simulink model "signal_tranmission"  (R2024b)
settings: Solver=ode45  StartTime=0.0  StopTime=10  FixedStep=0.000125  RelTol=1e-3
libraries: dspfdesign x500, commchan3 x1
(part 6 of 7)

== system signal_tranmission/SSB Modulator21/Balanced Modulator ==
  note: -S2(t)
  note: S1(t)
  note: -m(t)
  note: m(t)
  note: S2(t)
  note: S1(t)
  Input Signal : Inport
  Carrier Signal : Inport  Port=2
  -S2(t) : Product
  Add : Sum
  Add1 : Sum
  Add2 : Sum
  Constant : Constant
  Constant1 : Constant  Value=-1
  Constant2 : Constant
  Constant3 : Constant  Value=-1
  Product1 : Product
  S1(t) : Product
  S2(t) : Product
  DSBSC : Outport
  wires:
  Product1/1 -> Add1/1
  Add/1 -> S1(t)/1
  Constant3/1 -> -S2(t)/2
  Constant2/1 -> Add1/2
  S2(t)/1 -> -S2(t)/1
  Carrier Signal/1 -> S1(t)/2, S2(t)/1
  Constant/1 -> Add/2
  Add1/1 -> S2(t)/2
  Constant1/1 -> Product1/2
  -S2(t)/1 -> Add2/2
  S1(t)/1 -> Add2/1
  Input Signal/1 -> Product1/1, Add/1
  Add2/1 -> DSBSC/1

== system signal_tranmission/SSB Modulator22/Balanced Modulator ==
  note: -S2(t)
  note: S1(t)
  note: -m(t)
  note: m(t)
  note: S2(t)
  note: S1(t)
  Input Signal : Inport
  Carrier Signal : Inport  Port=2
  -S2(t) : Product
  Add : Sum
  Add1 : Sum
  Add2 : Sum
  Constant : Constant
  Constant1 : Constant  Value=-1
  Constant2 : Constant
  Constant3 : Constant  Value=-1
  Product1 : Product
  S1(t) : Product
  S2(t) : Product
  DSBSC : Outport
  wires:
  Product1/1 -> Add1/1
  Add/1 -> S1(t)/1
  Constant3/1 -> -S2(t)/2
  Constant2/1 -> Add1/2
  S2(t)/1 -> -S2(t)/1
  Carrier Signal/1 -> S1(t)/2, S2(t)/1
  Constant/1 -> Add/2
  Add1/1 -> S2(t)/2
  Constant1/1 -> Product1/2
  -S2(t)/1 -> Add2/2
  S1(t)/1 -> Add2/1
  Input Signal/1 -> Product1/1, Add/1
  Add2/1 -> DSBSC/1

== system signal_tranmission/SSB Modulator23/Balanced Modulator ==
  note: -S2(t)
  note: S1(t)
  note: -m(t)
  note: m(t)
  note: S2(t)
  note: S1(t)
  Input Signal : Inport
  Carrier Signal : Inport  Port=2
  -S2(t) : Product
  Add : Sum
  Add1 : Sum
  Add2 : Sum
  Constant : Constant
  Constant1 : Constant  Value=-1
  Constant2 : Constant
  Constant3 : Constant  Value=-1
  Product1 : Product
  S1(t) : Product
  S2(t) : Product
  DSBSC : Outport
  wires:
  Product1/1 -> Add1/1
  Add/1 -> S1(t)/1
  Constant3/1 -> -S2(t)/2
  Constant2/1 -> Add1/2
  S2(t)/1 -> -S2(t)/1
  Carrier Signal/1 -> S1(t)/2, S2(t)/1
  Constant/1 -> Add/2
  Add1/1 -> S2(t)/2
  Constant1/1 -> Product1/2
  -S2(t)/1 -> Add2/2
  S1(t)/1 -> Add2/1
  Input Signal/1 -> Product1/1, Add/1
  Add2/1 -> DSBSC/1

== system signal_tranmission/SSB Modulator24/Balanced Modulator ==
  note: -S2(t)
  note: S1(t)
  note: -m(t)
  note: m(t)
  note: S2(t)
  note: S1(t)
  Input Signal : Inport
  Carrier Signal : Inport  Port=2
  -S2(t) : Product
  Add : Sum
  Add1 : Sum
  Add2 : Sum
  Constant : Constant
  Constant1 : Constant  Value=-1
  Constant2 : Constant
  Constant3 : Constant  Value=-1
  Product1 : Product
  S1(t) : Product
  S2(t) : Product
  DSBSC : Outport
  wires:
  Product1/1 -> Add1/1
  Add/1 -> S1(t)/1
  Constant3/1 -> -S2(t)/2
  Constant2/1 -> Add1/2
  S2(t)/1 -> -S2(t)/1
  Carrier Signal/1 -> S1(t)/2, S2(t)/1
  Constant/1 -> Add/2
  Add1/1 -> S2(t)/2
  Constant1/1 -> Product1/2
  -S2(t)/1 -> Add2/2
  S1(t)/1 -> Add2/1
  Input Signal/1 -> Product1/1, Add/1
  Add2/1 -> DSBSC/1

== system signal_tranmission/SSB Modulator25/Balanced Modulator ==
  note: -S2(t)
  note: S1(t)
  note: -m(t)
  note: m(t)
  note: S2(t)
  note: S1(t)
  Input Signal : Inport
  Carrier Signal : Inport  Port=2
  -S2(t) : Product
  Add : Sum
  Add1 : Sum
  Add2 : Sum
  Constant : Constant
  Constant1 : Constant  Value=-1
  Constant2 : Constant
  Constant3 : Constant  Value=-1
  Product1 : Product
  S1(t) : Product
  S2(t) : Product
  DSBSC : Outport
  wires:
  Product1/1 -> Add1/1
  Add/1 -> S1(t)/1
  Constant3/1 -> -S2(t)/2
  Constant2/1 -> Add1/2
  S2(t)/1 -> -S2(t)/1
  Carrier Signal/1 -> S1(t)/2, S2(t)/1
  Constant/1 -> Add/2
  Add1/1 -> S2(t)/2
  Constant1/1 -> Product1/2
  -S2(t)/1 -> Add2/2
  S1(t)/1 -> Add2/1
  Input Signal/1 -> Product1/1, Add/1
  Add2/1 -> DSBSC/1

== system signal_tranmission/SSB Modulator26/Balanced Modulator ==
  note: -S2(t)
  note: S1(t)
  note: -m(t)
  note: m(t)
  note: S2(t)
  note: S1(t)
  Input Signal : Inport
  Carrier Signal : Inport  Port=2
  -S2(t) : Product
  Add : Sum
  Add1 : Sum
  Add2 : Sum
  Constant : Constant
  Constant1 : Constant  Value=-1
  Constant2 : Constant
  Constant3 : Constant  Value=-1
  Product1 : Product
  S1(t) : Product
  S2(t) : Product
  DSBSC : Outport
  wires:
  Product1/1 -> Add1/1
  Add/1 -> S1(t)/1
  Constant3/1 -> -S2(t)/2
  Constant2/1 -> Add1/2
  S2(t)/1 -> -S2(t)/1
  Carrier Signal/1 -> S1(t)/2, S2(t)/1
  Constant/1 -> Add/2
  Add1/1 -> S2(t)/2
  Constant1/1 -> Product1/2
  -S2(t)/1 -> Add2/2
  S1(t)/1 -> Add2/1
  Input Signal/1 -> Product1/1, Add/1
  Add2/1 -> DSBSC/1

== system signal_tranmission/SSB Modulator27/Balanced Modulator ==
  note: -S2(t)
  note: S1(t)
  note: -m(t)
  note: m(t)
  note: S2(t)
  note: S1(t)
  Input Signal : Inport
  Carrier Signal : Inport  Port=2
  -S2(t) : Product
  Add : Sum
  Add1 : Sum
  Add2 : Sum
  Constant : Constant
  Constant1 : Constant  Value=-1
  Constant2 : Constant
  Constant3 : Constant  Value=-1
  Product1 : Product
  S1(t) : Product
  S2(t) : Product
  DSBSC : Outport
  wires:
  Product1/1 -> Add1/1
  Add/1 -> S1(t)/1
  Constant3/1 -> -S2(t)/2
  Constant2/1 -> Add1/2
  S2(t)/1 -> -S2(t)/1
  Carrier Signal/1 -> S1(t)/2, S2(t)/1
  Constant/1 -> Add/2
  Add1/1 -> S2(t)/2
  Constant1/1 -> Product1/2
  -S2(t)/1 -> Add2/2
  S1(t)/1 -> Add2/1
  Input Signal/1 -> Product1/1, Add/1
  Add2/1 -> DSBSC/1

== system signal_tranmission/SSB Modulator28/Balanced Modulator ==
  note: -S2(t)
  note: S1(t)
  note: -m(t)
  note: m(t)
  note: S2(t)
  note: S1(t)
  Input Signal : Inport
  Carrier Signal : Inport  Port=2
  -S2(t) : Product
  Add : Sum
  Add1 : Sum
  Add2 : Sum
  Constant : Constant
  Constant1 : Constant  Value=-1
  Constant2 : Constant
  Constant3 : Constant  Value=-1
  Product1 : Product
  S1(t) : Product
  S2(t) : Product
  DSBSC : Outport
  wires:
  Product1/1 -> Add1/1
  Add/1 -> S1(t)/1
  Constant3/1 -> -S2(t)/2
  Constant2/1 -> Add1/2
  S2(t)/1 -> -S2(t)/1
  Carrier Signal/1 -> S1(t)/2, S2(t)/1
  Constant/1 -> Add/2
  Add1/1 -> S2(t)/2
  Constant1/1 -> Product1/2
  -S2(t)/1 -> Add2/2
  S1(t)/1 -> Add2/1
  Input Signal/1 -> Product1/1, Add/1
  Add2/1 -> DSBSC/1

== system signal_tranmission/SSB Modulator29/Balanced Modulator ==
  note: -S2(t)
  note: S1(t)
  note: -m(t)
  note: m(t)
  note: S2(t)
  note: S1(t)
  Input Signal : Inport
  Carrier Signal : Inport  Port=2
  -S2(t) : Product
  Add : Sum
  Add1 : Sum
  Add2 : Sum
  Constant : Constant
  Constant1 : Constant  Value=-1
  Constant2 : Constant
  Constant3 : Constant  Value=-1
  Product1 : Product
  S1(t) : Product
  S2(t) : Product
  DSBSC : Outport
  wires:
  Product1/1 -> Add1/1
  Add/1 -> S1(t)/1
  Constant3/1 -> -S2(t)/2
  Constant2/1 -> Add1/2
  S2(t)/1 -> -S2(t)/1
  Carrier Signal/1 -> S1(t)/2, S2(t)/1
  Constant/1 -> Add/2
  Add1/1 -> S2(t)/2
  Constant1/1 -> Product1/2
  -S2(t)/1 -> Add2/2
  S1(t)/1 -> Add2/1
  Input Signal/1 -> Product1/1, Add/1
  Add2/1 -> DSBSC/1

== system signal_tranmission/SSB Modulator3/Balanced Modulator ==
  note: -S2(t)
  note: S1(t)
  note: -m(t)
  note: m(t)
  note: S2(t)
  note: S1(t)
  Input Signal : Inport
  Carrier Signal : Inport  Port=2
  -S2(t) : Product
  Add : Sum
  Add1 : Sum
  Add2 : Sum
  Constant : Constant
  Constant1 : Constant  Value=-1
  Constant2 : Constant
  Constant3 : Constant  Value=-1
  Product1 : Product
  S1(t) : Product
  S2(t) : Product
  DSBSC : Outport
  wires:
  Product1/1 -> Add1/1
  Add/1 -> S1(t)/1
  Constant3/1 -> -S2(t)/2
  Constant2/1 -> Add1/2
  S2(t)/1 -> -S2(t)/1
  Carrier Signal/1 -> S1(t)/2, S2(t)/1
  Constant/1 -> Add/2
  Add1/1 -> S2(t)/2
  Constant1/1 -> Product1/2
  -S2(t)/1 -> Add2/2
  S1(t)/1 -> Add2/1
  Input Signal/1 -> Product1/1, Add/1
  Add2/1 -> DSBSC/1

== system signal_tranmission/SSB Modulator30/Balanced Modulator ==
  note: -S2(t)
  note: S1(t)
  note: -m(t)
  note: m(t)
  note: S2(t)
  note: S1(t)
  Input Signal : Inport
  Carrier Signal : Inport  Port=2
  -S2(t) : Product
  Add : Sum
  Add1 : Sum
  Add2 : Sum
  Constant : Constant
  Constant1 : Constant  Value=-1
  Constant2 : Constant
  Constant3 : Constant  Value=-1
  Product1 : Product
  S1(t) : Product
  S2(t) : Product
  DSBSC : Outport
  wires:
  Product1/1 -> Add1/1
  Add/1 -> S1(t)/1
  Constant3/1 -> -S2(t)/2
  Constant2/1 -> Add1/2
  S2(t)/1 -> -S2(t)/1
  Carrier Signal/1 -> S1(t)/2, S2(t)/1
  Constant/1 -> Add/2
  Add1/1 -> S2(t)/2
  Constant1/1 -> Product1/2
  -S2(t)/1 -> Add2/2
  S1(t)/1 -> Add2/1
  Input Signal/1 -> Product1/1, Add/1
  Add2/1 -> DSBSC/1

== system signal_tranmission/SSB Modulator31/Balanced Modulator ==
  note: -S2(t)
  note: S1(t)
  note: -m(t)
  note: m(t)
  note: S2(t)
  note: S1(t)
  Input Signal : Inport
  Carrier Signal : Inport  Port=2
  -S2(t) : Product
  Add : Sum
  Add1 : Sum
  Add2 : Sum
  Constant : Constant
  Constant1 : Constant  Value=-1
  Constant2 : Constant
  Constant3 : Constant  Value=-1
  Product1 : Product
  S1(t) : Product
  S2(t) : Product
  DSBSC : Outport
  wires:
  Product1/1 -> Add1/1
  Add/1 -> S1(t)/1
  Constant3/1 -> -S2(t)/2
  Constant2/1 -> Add1/2
  S2(t)/1 -> -S2(t)/1
  Carrier Signal/1 -> S1(t)/2, S2(t)/1
  Constant/1 -> Add/2
  Add1/1 -> S2(t)/2
  Constant1/1 -> Product1/2
  -S2(t)/1 -> Add2/2
  S1(t)/1 -> Add2/1
  Input Signal/1 -> Product1/1, Add/1
  Add2/1 -> DSBSC/1

== system signal_tranmission/SSB Modulator32/Balanced Modulator ==
  note: -S2(t)
  note: S1(t)
  note: -m(t)
  note: m(t)
  note: S2(t)
  note: S1(t)
  Input Signal : Inport
  Carrier Signal : Inport  Port=2
  -S2(t) : Product
  Add : Sum
  Add1 : Sum
  Add2 : Sum
  Constant : Constant
  Constant1 : Constant  Value=-1
  Constant2 : Constant
  Constant3 : Constant  Value=-1
  Product1 : Product
  S1(t) : Product
  S2(t) : Product
  DSBSC : Outport
  wires:
  Product1/1 -> Add1/1
  Add/1 -> S1(t)/1
  Constant3/1 -> -S2(t)/2
  Constant2/1 -> Add1/2
  S2(t)/1 -> -S2(t)/1
  Carrier Signal/1 -> S1(t)/2, S2(t)/1
  Constant/1 -> Add/2
  Add1/1 -> S2(t)/2
  Constant1/1 -> Product1/2
  -S2(t)/1 -> Add2/2
  S1(t)/1 -> Add2/1
  Input Signal/1 -> Product1/1, Add/1
  Add2/1 -> DSBSC/1

== system signal_tranmission/SSB Modulator33/Balanced Modulator ==
  note: -S2(t)
  note: S1(t)
  note: -m(t)
  note: m(t)
  note: S2(t)
  note: S1(t)
  Input Signal : Inport
  Carrier Signal : Inport  Port=2
  -S2(t) : Product
  Add : Sum
  Add1 : Sum
  Add2 : Sum
  Constant : Constant
  Constant1 : Constant  Value=-1
  Constant2 : Constant
  Constant3 : Constant  Value=-1
  Product1 : Product
  S1(t) : Product
  S2(t) : Product
  DSBSC : Outport
  wires:
  Product1/1 -> Add1/1
  Add/1 -> S1(t)/1
  Constant3/1 -> -S2(t)/2
  Constant2/1 -> Add1/2
  S2(t)/1 -> -S2(t)/1
  Carrier Signal/1 -> S1(t)/2, S2(t)/1
  Constant/1 -> Add/2
  Add1/1 -> S2(t)/2
  Constant1/1 -> Product1/2
  -S2(t)/1 -> Add2/2
  S1(t)/1 -> Add2/1
  Input Signal/1 -> Product1/1, Add/1
  Add2/1 -> DSBSC/1

== system signal_tranmission/SSB Modulator34/Balanced Modulator ==
  note: -S2(t)
  note: S1(t)
  note: -m(t)
  note: m(t)
  note: S2(t)
  note: S1(t)
  Input Signal : Inport
  Carrier Signal : Inport  Port=2
  -S2(t) : Product
  Add : Sum
  Add1 : Sum
  Add2 : Sum
  Constant : Constant
  Constant1 : Constant  Value=-1
  Constant2 : Constant
  Constant3 : Constant  Value=-1
  Product1 : Product
  S1(t) : Product
  S2(t) : Product
  DSBSC : Outport
  wires:
  Product1/1 -> Add1/1
  Add/1 -> S1(t)/1
  Constant3/1 -> -S2(t)/2
  Constant2/1 -> Add1/2
  S2(t)/1 -> -S2(t)/1
  Carrier Signal/1 -> S1(t)/2, S2(t)/1
  Constant/1 -> Add/2
  Add1/1 -> S2(t)/2
  Constant1/1 -> Product1/2
  -S2(t)/1 -> Add2/2
  S1(t)/1 -> Add2/1
  Input Signal/1 -> Product1/1, Add/1
  Add2/1 -> DSBSC/1

== system signal_tranmission/SSB Modulator35/Balanced Modulator ==
  note: -S2(t)
  note: S1(t)
  note: -m(t)
  note: m(t)
  note: S2(t)
  note: S1(t)
  Input Signal : Inport
  Carrier Signal : Inport  Port=2
  -S2(t) : Product
  Add : Sum
  Add1 : Sum
  Add2 : Sum
  Constant : Constant
  Constant1 : Constant  Value=-1
  Constant2 : Constant
  Constant3 : Constant  Value=-1
  Product1 : Product
  S1(t) : Product
  S2(t) : Product
  DSBSC : Outport
  wires:
  Product1/1 -> Add1/1
  Add/1 -> S1(t)/1
  Constant3/1 -> -S2(t)/2
  Constant2/1 -> Add1/2
  S2(t)/1 -> -S2(t)/1
  Carrier Signal/1 -> S1(t)/2, S2(t)/1
  Constant/1 -> Add/2
  Add1/1 -> S2(t)/2
  Constant1/1 -> Product1/2
  -S2(t)/1 -> Add2/2
  S1(t)/1 -> Add2/1
  Input Signal/1 -> Product1/1, Add/1
  Add2/1 -> DSBSC/1

== system signal_tranmission/SSB Modulator36/Balanced Modulator ==
  note: -S2(t)
  note: S1(t)
  note: -m(t)
  note: m(t)
  note: S2(t)
  note: S1(t)
  Input Signal : Inport
  Carrier Signal : Inport  Port=2
  -S2(t) : Product
  Add : Sum
  Add1 : Sum
  Add2 : Sum
  Constant : Constant
  Constant1 : Constant  Value=-1
  Constant2 : Constant
  Constant3 : Constant  Value=-1
  Product1 : Product
  S1(t) : Product
  S2(t) : Product
  DSBSC : Outport
  wires:
  Product1/1 -> Add1/1
  Add/1 -> S1(t)/1
  Constant3/1 -> -S2(t)/2
  Constant2/1 -> Add1/2
  S2(t)/1 -> -S2(t)/1
  Carrier Signal/1 -> S1(t)/2, S2(t)/1
  Constant/1 -> Add/2
  Add1/1 -> S2(t)/2
  Constant1/1 -> Product1/2
  -S2(t)/1 -> Add2/2
  S1(t)/1 -> Add2/1
  Input Signal/1 -> Product1/1, Add/1
  Add2/1 -> DSBSC/1

== system signal_tranmission/SSB Modulator37/Balanced Modulator ==
  note: -S2(t)
  note: S1(t)
  note: -m(t)
  note: m(t)
  note: S2(t)
  note: S1(t)
  Input Signal : Inport
  Carrier Signal : Inport  Port=2
  -S2(t) : Product
  Add : Sum
  Add1 : Sum
  Add2 : Sum
  Constant : Constant
  Constant1 : Constant  Value=-1
  Constant2 : Constant
  Constant3 : Constant  Value=-1
  Product1 : Product
  S1(t) : Product
  S2(t) : Product
  DSBSC : Outport
  wires:
  Product1/1 -> Add1/1
  Add/1 -> S1(t)/1
  Constant3/1 -> -S2(t)/2
  Constant2/1 -> Add1/2
  S2(t)/1 -> -S2(t)/1
  Carrier Signal/1 -> S1(t)/2, S2(t)/1
  Constant/1 -> Add/2
  Add1/1 -> S2(t)/2
  Constant1/1 -> Product1/2
  -S2(t)/1 -> Add2/2
  S1(t)/1 -> Add2/1
  Input Signal/1 -> Product1/1, Add/1
  Add2/1 -> DSBSC/1

== system signal_tranmission/SSB Modulator38/Balanced Modulator ==
  note: -S2(t)
  note: S1(t)
  note: -m(t)
  note: m(t)
  note: S2(t)
  note: S1(t)
  Input Signal : Inport
  Carrier Signal : Inport  Port=2
  -S2(t) : Product
  Add : Sum
  Add1 : Sum
  Add2 : Sum
  Constant : Constant
  Constant1 : Constant  Value=-1
  Constant2 : Constant
  Constant3 : Constant  Value=-1
  Product1 : Product
  S1(t) : Product
  S2(t) : Product
  DSBSC : Outport
  wires:
  Product1/1 -> Add1/1
  Add/1 -> S1(t)/1
  Constant3/1 -> -S2(t)/2
  Constant2/1 -> Add1/2
  S2(t)/1 -> -S2(t)/1
  Carrier Signal/1 -> S1(t)/2, S2(t)/1
  Constant/1 -> Add/2
  Add1/1 -> S2(t)/2
  Constant1/1 -> Product1/2
  -S2(t)/1 -> Add2/2
  S1(t)/1 -> Add2/1
  Input Signal/1 -> Product1/1, Add/1
  Add2/1 -> DSBSC/1

== system signal_tranmission/SSB Modulator39/Balanced Modulator ==
  note: -S2(t)
  note: S1(t)
  note: -m(t)
  note: m(t)
  note: S2(t)
  note: S1(t)
  Input Signal : Inport
  Carrier Signal : Inport  Port=2
  -S2(t) : Product
  Add : Sum
  Add1 : Sum
  Add2 : Sum
  Constant : Constant
  Constant1 : Constant  Value=-1
  Constant2 : Constant
  Constant3 : Constant  Value=-1
  Product1 : Product
  S1(t) : Product
  S2(t) : Product
  DSBSC : Outport
  wires:
  Product1/1 -> Add1/1
  Add/1 -> S1(t)/1
  Constant3/1 -> -S2(t)/2
  Constant2/1 -> Add1/2
  S2(t)/1 -> -S2(t)/1
  Carrier Signal/1 -> S1(t)/2, S2(t)/1
  Constant/1 -> Add/2
  Add1/1 -> S2(t)/2
  Constant1/1 -> Product1/2
  -S2(t)/1 -> Add2/2
  S1(t)/1 -> Add2/1
  Input Signal/1 -> Product1/1, Add/1
  Add2/1 -> DSBSC/1

== system signal_tranmission/SSB Modulator4/Balanced Modulator ==
  note: -S2(t)
  note: S1(t)
  note: -m(t)
  note: m(t)
  note: S2(t)
  note: S1(t)
  Input Signal : Inport
  Carrier Signal : Inport  Port=2
  -S2(t) : Product
  Add : Sum
  Add1 : Sum
  Add2 : Sum
  Constant : Constant
  Constant1 : Constant  Value=-1
  Constant2 : Constant
  Constant3 : Constant  Value=-1
  Product1 : Product
  S1(t) : Product
  S2(t) : Product
  DSBSC : Outport
  wires:
  Product1/1 -> Add1/1
  Add/1 -> S1(t)/1
  Constant3/1 -> -S2(t)/2
  Constant2/1 -> Add1/2
  S2(t)/1 -> -S2(t)/1
  Carrier Signal/1 -> S1(t)/2, S2(t)/1
  Constant/1 -> Add/2
  Add1/1 -> S2(t)/2
  Constant1/1 -> Product1/2
  -S2(t)/1 -> Add2/2
  S1(t)/1 -> Add2/1
  Input Signal/1 -> Product1/1, Add/1
  Add2/1 -> DSBSC/1

== system signal_tranmission/SSB Modulator40/Balanced Modulator ==
  note: -S2(t)
  note: S1(t)
  note: -m(t)
  note: m(t)
  note: S2(t)
  note: S1(t)
  Input Signal : Inport
  Carrier Signal : Inport  Port=2
  -S2(t) : Product
  Add : Sum
  Add1 : Sum
  Add2 : Sum
  Constant : Constant
  Constant1 : Constant  Value=-1
  Constant2 : Constant
  Constant3 : Constant  Value=-1
  Product1 : Product
  S1(t) : Product
  S2(t) : Product
  DSBSC : Outport
  wires:
  Product1/1 -> Add1/1
  Add/1 -> S1(t)/1
  Constant3/1 -> -S2(t)/2
  Constant2/1 -> Add1/2
  S2(t)/1 -> -S2(t)/1
  Carrier Signal/1 -> S1(t)/2, S2(t)/1
  Constant/1 -> Add/2
  Add1/1 -> S2(t)/2
  Constant1/1 -> Product1/2
  -S2(t)/1 -> Add2/2
  S1(t)/1 -> Add2/1
  Input Signal/1 -> Product1/1, Add/1
  Add2/1 -> DSBSC/1

== system signal_tranmission/SSB Modulator41/Balanced Modulator ==
  note: -S2(t)
  note: S1(t)
  note: -m(t)
  note: m(t)
  note: S2(t)
  note: S1(t)
  Input Signal : Inport
  Carrier Signal : Inport  Port=2
  -S2(t) : Product
  Add : Sum
  Add1 : Sum
  Add2 : Sum
  Constant : Constant
  Constant1 : Constant  Value=-1
  Constant2 : Constant
  Constant3 : Constant  Value=-1
  Product1 : Product
  S1(t) : Product
  S2(t) : Product
  DSBSC : Outport
  wires:
  Product1/1 -> Add1/1
  Add/1 -> S1(t)/1
  Constant3/1 -> -S2(t)/2
  Constant2/1 -> Add1/2
  S2(t)/1 -> -S2(t)/1
  Carrier Signal/1 -> S1(t)/2, S2(t)/1
  Constant/1 -> Add/2
  Add1/1 -> S2(t)/2
  Constant1/1 -> Product1/2
  -S2(t)/1 -> Add2/2
  S1(t)/1 -> Add2/1
  Input Signal/1 -> Product1/1, Add/1
  Add2/1 -> DSBSC/1

== system signal_tranmission/SSB Modulator42/Balanced Modulator ==
  note: -S2(t)
  note: S1(t)
  note: -m(t)
  note: m(t)
  note: S2(t)
  note: S1(t)
  Input Signal : Inport
  Carrier Signal : Inport  Port=2
  -S2(t) : Product
  Add : Sum
  Add1 : Sum
  Add2 : Sum
  Constant : Constant
  Constant1 : Constant  Value=-1
  Constant2 : Constant
  Constant3 : Constant  Value=-1
  Product1 : Product
  S1(t) : Product
  S2(t) : Product
  DSBSC : Outport
  wires:
  Product1/1 -> Add1/1
  Add/1 -> S1(t)/1
  Constant3/1 -> -S2(t)/2
  Constant2/1 -> Add1/2
  S2(t)/1 -> -S2(t)/1
  Carrier Signal/1 -> S1(t)/2, S2(t)/1
  Constant/1 -> Add/2
  Add1/1 -> S2(t)/2
  Constant1/1 -> Product1/2
  -S2(t)/1 -> Add2/2
  S1(t)/1 -> Add2/1
  Input Signal/1 -> Product1/1, Add/1
  Add2/1 -> DSBSC/1

== system signal_tranmission/SSB Modulator43/Balanced Modulator ==
  note: -S2(t)
  note: S1(t)
  note: -m(t)
  note: m(t)
  note: S2(t)
  note: S1(t)
  Input Signal : Inport
  Carrier Signal : Inport  Port=2
  -S2(t) : Product
  Add : Sum
  Add1 : Sum
  Add2 : Sum
  Constant : Constant
  Constant1 : Constant  Value=-1
  Constant2 : Constant
  Constant3 : Constant  Value=-1
  Product1 : Product
  S1(t) : Product
  S2(t) : Product
  DSBSC : Outport
  wires:
  Product1/1 -> Add1/1
  Add/1 -> S1(t)/1
  Constant3/1 -> -S2(t)/2
  Constant2/1 -> Add1/2
  S2(t)/1 -> -S2(t)/1
  Carrier Signal/1 -> S1(t)/2, S2(t)/1
  Constant/1 -> Add/2
  Add1/1 -> S2(t)/2
  Constant1/1 -> Product1/2
  -S2(t)/1 -> Add2/2
  S1(t)/1 -> Add2/1
  Input Signal/1 -> Product1/1, Add/1
  Add2/1 -> DSBSC/1

== system signal_tranmission/SSB Modulator44/Balanced Modulator ==
  note: -S2(t)
  note: S1(t)
  note: -m(t)
  note: m(t)
  note: S2(t)
  note: S1(t)
  Input Signal : Inport
  Carrier Signal : Inport  Port=2
  -S2(t) : Product
  Add : Sum
  Add1 : Sum
  Add2 : Sum
  Constant : Constant
  Constant1 : Constant  Value=-1
  Constant2 : Constant
  Constant3 : Constant  Value=-1
  Product1 : Product
  S1(t) : Product
  S2(t) : Product
  DSBSC : Outport
  wires:
  Product1/1 -> Add1/1
  Add/1 -> S1(t)/1
  Constant3/1 -> -S2(t)/2
  Constant2/1 -> Add1/2
  S2(t)/1 -> -S2(t)/1
  Carrier Signal/1 -> S1(t)/2, S2(t)/1
  Constant/1 -> Add/2
  Add1/1 -> S2(t)/2
  Constant1/1 -> Product1/2
  -S2(t)/1 -> Add2/2
  S1(t)/1 -> Add2/1
  Input Signal/1 -> Product1/1, Add/1
  Add2/1 -> DSBSC/1

== system signal_tranmission/SSB Modulator45/Balanced Modulator ==
  note: -S2(t)
  note: S1(t)
  note: -m(t)
  note: m(t)
  note: S2(t)
  note: S1(t)
  Input Signal : Inport
  Carrier Signal : Inport  Port=2
  -S2(t) : Product
  Add : Sum
  Add1 : Sum
  Add2 : Sum
  Constant : Constant
  Constant1 : Constant  Value=-1
  Constant2 : Constant
  Constant3 : Constant  Value=-1
  Product1 : Product
  S1(t) : Product
  S2(t) : Product
  DSBSC : Outport
  wires:
  Product1/1 -> Add1/1
  Add/1 -> S1(t)/1
  Constant3/1 -> -S2(t)/2
  Constant2/1 -> Add1/2
  S2(t)/1 -> -S2(t)/1
  Carrier Signal/1 -> S1(t)/2, S2(t)/1
  Constant/1 -> Add/2
  Add1/1 -> S2(t)/2
  Constant1/1 -> Product1/2
  -S2(t)/1 -> Add2/2
  S1(t)/1 -> Add2/1
  Input Signal/1 -> Product1/1, Add/1
  Add2/1 -> DSBSC/1

== system signal_tranmission/SSB Modulator46/Balanced Modulator ==
  note: -S2(t)
  note: S1(t)
  note: -m(t)
  note: m(t)
  note: S2(t)
  note: S1(t)
  Input Signal : Inport
  Carrier Signal : Inport  Port=2
  -S2(t) : Product
  Add : Sum
  Add1 : Sum
  Add2 : Sum
  Constant : Constant
  Constant1 : Constant  Value=-1
  Constant2 : Constant
  Constant3 : Constant  Value=-1
  Product1 : Product
  S1(t) : Product
  S2(t) : Product
  DSBSC : Outport
  wires:
  Product1/1 -> Add1/1
  Add/1 -> S1(t)/1
  Constant3/1 -> -S2(t)/2
  Constant2/1 -> Add1/2
  S2(t)/1 -> -S2(t)/1
  Carrier Signal/1 -> S1(t)/2, S2(t)/1
  Constant/1 -> Add/2
  Add1/1 -> S2(t)/2
  Constant1/1 -> Product1/2
  -S2(t)/1 -> Add2/2
  S1(t)/1 -> Add2/1
  Input Signal/1 -> Product1/1, Add/1
  Add2/1 -> DSBSC/1

== system signal_tranmission/SSB Modulator47/Balanced Modulator ==
  note: -S2(t)
  note: S1(t)
  note: -m(t)
  note: m(t)
  note: S2(t)
  note: S1(t)
  Input Signal : Inport
  Carrier Signal : Inport  Port=2
  -S2(t) : Product
  Add : Sum
  Add1 : Sum
  Add2 : Sum
  Constant : Constant
  Constant1 : Constant  Value=-1
  Constant2 : Constant
  Constant3 : Constant  Value=-1
  Product1 : Product
  S1(t) : Product
  S2(t) : Product
  DSBSC : Outport
  wires:
  Product1/1 -> Add1/1
  Add/1 -> S1(t)/1
  Constant3/1 -> -S2(t)/2
  Constant2/1 -> Add1/2
  S2(t)/1 -> -S2(t)/1
  Carrier Signal/1 -> S1(t)/2, S2(t)/1
  Constant/1 -> Add/2
  Add1/1 -> S2(t)/2
  Constant1/1 -> Product1/2
  -S2(t)/1 -> Add2/2
  S1(t)/1 -> Add2/1
  Input Signal/1 -> Product1/1, Add/1
  Add2/1 -> DSBSC/1

== system signal_tranmission/SSB Modulator48/Balanced Modulator ==
  note: -S2(t)
  note: S1(t)
  note: -m(t)
  note: m(t)
  note: S2(t)
  note: S1(t)
  Input Signal : Inport
  Carrier Signal : Inport  Port=2
  -S2(t) : Product
  Add : Sum
  Add1 : Sum
  Add2 : Sum
  Constant : Constant
  Constant1 : Constant  Value=-1
  Constant2 : Constant
  Constant3 : Constant  Value=-1
  Product1 : Product
  S1(t) : Product
  S2(t) : Product
  DSBSC : Outport
  wires:
  Product1/1 -> Add1/1
  Add/1 -> S1(t)/1
  Constant3/1 -> -S2(t)/2
  Constant2/1 -> Add1/2
  S2(t)/1 -> -S2(t)/1
  Carrier Signal/1 -> S1(t)/2, S2(t)/1
  Constant/1 -> Add/2
  Add1/1 -> S2(t)/2
  Constant1/1 -> Product1/2
  -S2(t)/1 -> Add2/2
  S1(t)/1 -> Add2/1
  Input Signal/1 -> Product1/1, Add/1
  Add2/1 -> DSBSC/1

== system signal_tranmission/SSB Modulator49/Balanced Modulator ==
  note: -S2(t)
  note: S1(t)
  note: -m(t)
  note: m(t)
  note: S2(t)
  note: S1(t)
  Input Signal : Inport
  Carrier Signal : Inport  Port=2
  -S2(t) : Product
  Add : Sum
  Add1 : Sum
  Add2 : Sum
  Constant : Constant
  Constant1 : Constant  Value=-1
  Constant2 : Constant
  Constant3 : Constant  Value=-1
  Product1 : Product
  S1(t) : Product
  S2(t) : Product
  DSBSC : Outport
  wires:
  Product1/1 -> Add1/1
  Add/1 -> S1(t)/1
  Constant3/1 -> -S2(t)/2
  Constant2/1 -> Add1/2
  S2(t)/1 -> -S2(t)/1
  Carrier Signal/1 -> S1(t)/2, S2(t)/1
  Constant/1 -> Add/2
  Add1/1 -> S2(t)/2
  Constant1/1 -> Product1/2
  -S2(t)/1 -> Add2/2
  S1(t)/1 -> Add2/1
  Input Signal/1 -> Product1/1, Add/1
  Add2/1 -> DSBSC/1

== system signal_tranmission/SSB Modulator5/Balanced Modulator ==
  note: -S2(t)
  note: S1(t)
  note: -m(t)
  note: m(t)
  note: S2(t)
  note: S1(t)
  Input Signal : Inport
  Carrier Signal : Inport  Port=2
  -S2(t) : Product
  Add : Sum
  Add1 : Sum
  Add2 : Sum
  Constant : Constant
  Constant1 : Constant  Value=-1
  Constant2 : Constant
  Constant3 : Constant  Value=-1
  Product1 : Product
  S1(t) : Product
  S2(t) : Product
  DSBSC : Outport
  wires:
  Product1/1 -> Add1/1
  Add/1 -> S1(t)/1
  Constant3/1 -> -S2(t)/2
  Constant2/1 -> Add1/2
  S2(t)/1 -> -S2(t)/1
  Carrier Signal/1 -> S1(t)/2, S2(t)/1
  Constant/1 -> Add/2
  Add1/1 -> S2(t)/2
  Constant1/1 -> Product1/2
  -S2(t)/1 -> Add2/2
  S1(t)/1 -> Add2/1
  Input Signal/1 -> Product1/1, Add/1
  Add2/1 -> DSBSC/1

== system signal_tranmission/SSB Modulator50/Balanced Modulator ==
  note: -S2(t)
  note: S1(t)
  note: -m(t)
  note: m(t)
  note: S2(t)
  note: S1(t)
  Input Signal : Inport
  Carrier Signal : Inport  Port=2
  -S2(t) : Product
  Add : Sum
  Add1 : Sum
  Add2 : Sum
  Constant : Constant
  Constant1 : Constant  Value=-1
  Constant2 : Constant
  Constant3 : Constant  Value=-1
  Product1 : Product
  S1(t) : Product
  S2(t) : Product
  DSBSC : Outport
  wires:
  Product1/1 -> Add1/1
  Add/1 -> S1(t)/1
  Constant3/1 -> -S2(t)/2
  Constant2/1 -> Add1/2
  S2(t)/1 -> -S2(t)/1
  Carrier Signal/1 -> S1(t)/2, S2(t)/1
  Constant/1 -> Add/2
  Add1/1 -> S2(t)/2
  Constant1/1 -> Product1/2
  -S2(t)/1 -> Add2/2
  S1(t)/1 -> Add2/1
  Input Signal/1 -> Product1/1, Add/1
  Add2/1 -> DSBSC/1

== system signal_tranmission/SSB Modulator51/Balanced Modulator ==
  note: -S2(t)
  note: S1(t)
  note: -m(t)
  note: m(t)
  note: S2(t)
  note: S1(t)
  Input Signal : Inport
  Carrier Signal : Inport  Port=2
  -S2(t) : Product
  Add : Sum
  Add1 : Sum
  Add2 : Sum
  Constant : Constant
  Constant1 : Constant  Value=-1
  Constant2 : Constant
  Constant3 : Constant  Value=-1
  Product1 : Product
  S1(t) : Product
  S2(t) : Product
  DSBSC : Outport
  wires:
  Product1/1 -> Add1/1
  Add/1 -> S1(t)/1
  Constant3/1 -> -S2(t)/2
  Constant2/1 -> Add1/2
  S2(t)/1 -> -S2(t)/1
  Carrier Signal/1 -> S1(t)/2, S2(t)/1
  Constant/1 -> Add/2
  Add1/1 -> S2(t)/2
  Constant1/1 -> Product1/2
  -S2(t)/1 -> Add2/2
  S1(t)/1 -> Add2/1
  Input Signal/1 -> Product1/1, Add/1
  Add2/1 -> DSBSC/1

== system signal_tranmission/SSB Modulator52/Balanced Modulator ==
  note: -S2(t)
  note: S1(t)
  note: -m(t)
  note: m(t)
  note: S2(t)
  note: S1(t)
  Input Signal : Inport
  Carrier Signal : Inport  Port=2
  -S2(t) : Product
  Add : Sum
  Add1 : Sum
  Add2 : Sum
  Constant : Constant
  Constant1 : Constant  Value=-1
  Constant2 : Constant
  Constant3 : Constant  Value=-1
  Product1 : Product
  S1(t) : Product
  S2(t) : Product
  DSBSC : Outport
  wires:
  Product1/1 -> Add1/1
  Add/1 -> S1(t)/1
  Constant3/1 -> -S2(t)/2
  Constant2/1 -> Add1/2
  S2(t)/1 -> -S2(t)/1
  Carrier Signal/1 -> S1(t)/2, S2(t)/1
  Constant/1 -> Add/2
  Add1/1 -> S2(t)/2
  Constant1/1 -> Product1/2
  -S2(t)/1 -> Add2/2
  S1(t)/1 -> Add2/1
  Input Signal/1 -> Product1/1, Add/1
  Add2/1 -> DSBSC/1

== system signal_tranmission/SSB Modulator53/Balanced Modulator ==
  note: -S2(t)
  note: S1(t)
  note: -m(t)
  note: m(t)
  note: S2(t)
  note: S1(t)
  Input Signal : Inport
  Carrier Signal : Inport  Port=2
  -S2(t) : Product
  Add : Sum
  Add1 : Sum
  Add2 : Sum
  Constant : Constant
  Constant1 : Constant  Value=-1
  Constant2 : Constant
  Constant3 : Constant  Value=-1
  Product1 : Product
  S1(t) : Product
  S2(t) : Product
  DSBSC : Outport
  wires:
  Product1/1 -> Add1/1
  Add/1 -> S1(t)/1
  Constant3/1 -> -S2(t)/2
  Constant2/1 -> Add1/2
  S2(t)/1 -> -S2(t)/1
  Carrier Signal/1 -> S1(t)/2, S2(t)/1
  Constant/1 -> Add/2
  Add1/1 -> S2(t)/2
  Constant1/1 -> Product1/2
  -S2(t)/1 -> Add2/2
  S1(t)/1 -> Add2/1
  Input Signal/1 -> Product1/1, Add/1
  Add2/1 -> DSBSC/1

== system signal_tranmission/SSB Modulator54/Balanced Modulator ==
  note: -S2(t)
  note: S1(t)
  note: -m(t)
  note: m(t)
  note: S2(t)
  note: S1(t)
  Input Signal : Inport
  Carrier Signal : Inport  Port=2
  -S2(t) : Product
  Add : Sum
  Add1 : Sum
  Add2 : Sum
  Constant : Constant
  Constant1 : Constant  Value=-1
  Constant2 : Constant
  Constant3 : Constant  Value=-1
  Product1 : Product
  S1(t) : Product
  S2(t) : Product
  DSBSC : Outport
  wires:
  Product1/1 -> Add1/1
  Add/1 -> S1(t)/1
  Constant3/1 -> -S2(t)/2
  Constant2/1 -> Add1/2
  S2(t)/1 -> -S2(t)/1
  Carrier Signal/1 -> S1(t)/2, S2(t)/1
  Constant/1 -> Add/2
  Add1/1 -> S2(t)/2
  Constant1/1 -> Product1/2
  -S2(t)/1 -> Add2/2
  S1(t)/1 -> Add2/1
  Input Signal/1 -> Product1/1, Add/1
  Add2/1 -> DSBSC/1

== system signal_tranmission/SSB Modulator55/Balanced Modulator ==
  note: -S2(t)
  note: S1(t)
  note: -m(t)
  note: m(t)
  note: S2(t)
  note: S1(t)
  Input Signal : Inport
  Carrier Signal : Inport  Port=2
  -S2(t) : Product
  Add : Sum
  Add1 : Sum
  Add2 : Sum
  Constant : Constant
  Constant1 : Constant  Value=-1
  Constant2 : Constant
  Constant3 : Constant  Value=-1
  Product1 : Product
  S1(t) : Product
  S2(t) : Product
  DSBSC : Outport
  wires:
  Product1/1 -> Add1/1
  Add/1 -> S1(t)/1
  Constant3/1 -> -S2(t)/2
  Constant2/1 -> Add1/2
  S2(t)/1 -> -S2(t)/1
  Carrier Signal/1 -> S1(t)/2, S2(t)/1
  Constant/1 -> Add/2
  Add1/1 -> S2(t)/2
  Constant1/1 -> Product1/2
  -S2(t)/1 -> Add2/2
  S1(t)/1 -> Add2/1
  Input Signal/1 -> Product1/1, Add/1
  Add2/1 -> DSBSC/1

== system signal_tranmission/SSB Modulator56/Balanced Modulator ==
  note: -S2(t)
  note: S1(t)
  note: -m(t)
  note: m(t)
  note: S2(t)
  note: S1(t)
  Input Signal : Inport
  Carrier Signal : Inport  Port=2
  -S2(t) : Product
  Add : Sum
  Add1 : Sum
  Add2 : Sum
  Constant : Constant
  Constant1 : Constant  Value=-1
  Constant2 : Constant
  Constant3 : Constant  Value=-1
  Product1 : Product
  S1(t) : Product
  S2(t) : Product
  DSBSC : Outport
  wires:
  Product1/1 -> Add1/1
  Add/1 -> S1(t)/1
  Constant3/1 -> -S2(t)/2
  Constant2/1 -> Add1/2
  S2(t)/1 -> -S2(t)/1
  Carrier Signal/1 -> S1(t)/2, S2(t)/1
  Constant/1 -> Add/2
  Add1/1 -> S2(t)/2
  Constant1/1 -> Product1/2
  -S2(t)/1 -> Add2/2
  S1(t)/1 -> Add2/1
  Input Signal/1 -> Product1/1, Add/1
  Add2/1 -> DSBSC/1

== system signal_tranmission/SSB Modulator57/Balanced Modulator ==
  note: -S2(t)
  note: S1(t)
  note: -m(t)
  note: m(t)
  note: S2(t)
  note: S1(t)
  Input Signal : Inport
  Carrier Signal : Inport  Port=2
  -S2(t) : Product
  Add : Sum
  Add1 : Sum
  Add2 : Sum
  Constant : Constant
  Constant1 : Constant  Value=-1
  Constant2 : Constant
  Constant3 : Constant  Value=-1
  Product1 : Product
  S1(t) : Product
  S2(t) : Product
  DSBSC : Outport
  wires:
  Product1/1 -> Add1/1
  Add/1 -> S1(t)/1
  Constant3/1 -> -S2(t)/2
  Constant2/1 -> Add1/2
  S2(t)/1 -> -S2(t)/1
  Carrier Signal/1 -> S1(t)/2, S2(t)/1
  Constant/1 -> Add/2
  Add1/1 -> S2(t)/2
  Constant1/1 -> Product1/2
  -S2(t)/1 -> Add2/2
  S1(t)/1 -> Add2/1
  Input Signal/1 -> Product1/1, Add/1
  Add2/1 -> DSBSC/1

== system signal_tranmission/SSB Modulator58/Balanced Modulator ==
  note: -S2(t)
  note: S1(t)
  note: -m(t)
  note: m(t)
  note: S2(t)
  note: S1(t)
  Input Signal : Inport
  Carrier Signal : Inport  Port=2
  -S2(t) : Product
  Add : Sum
  Add1 : Sum
  Add2 : Sum
  Constant : Constant
  Constant1 : Constant  Value=-1
  Constant2 : Constant
  Constant3 : Constant  Value=-1
  Product1 : Product
  S1(t) : Product
  S2(t) : Product
  DSBSC : Outport
  wires:
  Product1/1 -> Add1/1
  Add/1 -> S1(t)/1
  Constant3/1 -> -S2(t)/2
  Constant2/1 -> Add1/2
  S2(t)/1 -> -S2(t)/1
  Carrier Signal/1 -> S1(t)/2, S2(t)/1
  Constant/1 -> Add/2
  Add1/1 -> S2(t)/2
  Constant1/1 -> Product1/2
  -S2(t)/1 -> Add2/2
  S1(t)/1 -> Add2/1
  Input Signal/1 -> Product1/1, Add/1
  Add2/1 -> DSBSC/1

== system signal_tranmission/SSB Modulator59/Balanced Modulator ==
  note: -S2(t)
  note: S1(t)
  note: -m(t)
  note: m(t)
  note: S2(t)
  note: S1(t)
  Input Signal : Inport
  Carrier Signal : Inport  Port=2
  -S2(t) : Product
  Add : Sum
  Add1 : Sum
  Add2 : Sum
  Constant : Constant
  Constant1 : Constant  Value=-1
  Constant2 : Constant
  Constant3 : Constant  Value=-1
  Product1 : Product
  S1(t) : Product
  S2(t) : Product
  DSBSC : Outport
  wires:
  Product1/1 -> Add1/1
  Add/1 -> S1(t)/1
  Constant3/1 -> -S2(t)/2
  Constant2/1 -> Add1/2
  S2(t)/1 -> -S2(t)/1
  Carrier Signal/1 -> S1(t)/2, S2(t)/1
  Constant/1 -> Add/2
  Add1/1 -> S2(t)/2
  Constant1/1 -> Product1/2
  -S2(t)/1 -> Add2/2
  S1(t)/1 -> Add2/1
  Input Signal/1 -> Product1/1, Add/1
  Add2/1 -> DSBSC/1

== system signal_tranmission/SSB Modulator6/Balanced Modulator ==
  note: -S2(t)
  note: S1(t)
  note: -m(t)
  note: m(t)
  note: S2(t)
  note: S1(t)
  Input Signal : Inport
  Carrier Signal : Inport  Port=2
  -S2(t) : Product
  Add : Sum
  Add1 : Sum
  Add2 : Sum
  Constant : Constant
  Constant1 : Constant  Value=-1
  Constant2 : Constant
  Constant3 : Constant  Value=-1
  Product1 : Product
  S1(t) : Product
  S2(t) : Product
  DSBSC : Outport
  wires:
  Product1/1 -> Add1/1
  Add/1 -> S1(t)/1
  Constant3/1 -> -S2(t)/2
  Constant2/1 -> Add1/2
  S2(t)/1 -> -S2(t)/1
  Carrier Signal/1 -> S1(t)/2, S2(t)/1
  Constant/1 -> Add/2
  Add1/1 -> S2(t)/2
  Constant1/1 -> Product1/2
  -S2(t)/1 -> Add2/2
  S1(t)/1 -> Add2/1
  Input Signal/1 -> Product1/1, Add/1
  Add2/1 -> DSBSC/1

== system signal_tranmission/SSB Modulator60/Balanced Modulator ==
  note: -S2(t)
  note: S1(t)
  note: -m(t)
  note: m(t)
  note: S2(t)
  note: S1(t)
  Input Signal : Inport
  Carrier Signal : Inport  Port=2
  -S2(t) : Product
  Add : Sum
  Add1 : Sum
  Add2 : Sum
  Constant : Constant
  Constant1 : Constant  Value=-1
  Constant2 : Constant
  Constant3 : Constant  Value=-1
  Product1 : Product
  S1(t) : Product
  S2(t) : Product
  DSBSC : Outport
  wires:
  Product1/1 -> Add1/1
  Add/1 -> S1(t)/1
  Constant3/1 -> -S2(t)/2
  Constant2/1 -> Add1/2
  S2(t)/1 -> -S2(t)/1
  Carrier Signal/1 -> S1(t)/2, S2(t)/1
  Constant/1 -> Add/2
  Add1/1 -> S2(t)/2
  Constant1/1 -> Product1/2
  -S2(t)/1 -> Add2/2
  S1(t)/1 -> Add2/1
  Input Signal/1 -> Product1/1, Add/1
  Add2/1 -> DSBSC/1

== system signal_tranmission/SSB Modulator61/Balanced Modulator ==
  note: -S2(t)
  note: S1(t)
  note: -m(t)
  note: m(t)
  note: S2(t)
  note: S1(t)
  Input Signal : Inport
  Carrier Signal : Inport  Port=2
  -S2(t) : Product
  Add : Sum
  Add1 : Sum
  Add2 : Sum
  Constant : Constant
  Constant1 : Constant  Value=-1
  Constant2 : Constant
  Constant3 : Constant  Value=-1
  Product1 : Product
  S1(t) : Product
  S2(t) : Product
  DSBSC : Outport
  wires:
  Product1/1 -> Add1/1
  Add/1 -> S1(t)/1
  Constant3/1 -> -S2(t)/2
  Constant2/1 -> Add1/2
  S2(t)/1 -> -S2(t)/1
  Carrier Signal/1 -> S1(t)/2, S2(t)/1
  Constant/1 -> Add/2
  Add1/1 -> S2(t)/2
  Constant1/1 -> Product1/2
  -S2(t)/1 -> Add2/2
  S1(t)/1 -> Add2/1
  Input Signal/1 -> Product1/1, Add/1
  Add2/1 -> DSBSC/1

== system signal_tranmission/SSB Modulator62/Balanced Modulator ==
  note: -S2(t)
  note: S1(t)
  note: -m(t)
  note: m(t)
  note: S2(t)
  note: S1(t)
  Input Signal : Inport
  Carrier Signal : Inport  Port=2
  -S2(t) : Product
  Add : Sum
  Add1 : Sum
  Add2 : Sum
  Constant : Constant
  Constant1 : Constant  Value=-1
  Constant2 : Constant
  Constant3 : Constant  Value=-1
  Product1 : Product
  S1(t) : Product
  S2(t) : Product
  DSBSC : Outport
  wires:
  Product1/1 -> Add1/1
  Add/1 -> S1(t)/1
  Constant3/1 -> -S2(t)/2
  Constant2/1 -> Add1/2
  S2(t)/1 -> -S2(t)/1
  Carrier Signal/1 -> S1(t)/2, S2(t)/1
  Constant/1 -> Add/2
  Add1/1 -> S2(t)/2
  Constant1/1 -> Product1/2
  -S2(t)/1 -> Add2/2
  S1(t)/1 -> Add2/1
  Input Signal/1 -> Product1/1, Add/1
  Add2/1 -> DSBSC/1

== system signal_tranmission/SSB Modulator63/Balanced Modulator ==
  note: -S2(t)
  note: S1(t)
  note: -m(t)
  note: m(t)
  note: S2(t)
  note: S1(t)
  Input Signal : Inport
  Carrier Signal : Inport  Port=2
  -S2(t) : Product
  Add : Sum
  Add1 : Sum
  Add2 : Sum
  Constant : Constant
  Constant1 : Constant  Value=-1
  Constant2 : Constant
  Constant3 : Constant  Value=-1
  Product1 : Product
  S1(t) : Product
  S2(t) : Product
  DSBSC : Outport
  wires:
  Product1/1 -> Add1/1
  Add/1 -> S1(t)/1
  Constant3/1 -> -S2(t)/2
  Constant2/1 -> Add1/2
  S2(t)/1 -> -S2(t)/1
  Carrier Signal/1 -> S1(t)/2, S2(t)/1
  Constant/1 -> Add/2
  Add1/1 -> S2(t)/2
  Constant1/1 -> Product1/2
  -S2(t)/1 -> Add2/2
  S1(t)/1 -> Add2/1
  Input Signal/1 -> Product1/1, Add/1
  Add2/1 -> DSBSC/1

== system signal_tranmission/SSB Modulator64/Balanced Modulator ==
  note: -S2(t)
  note: S1(t)
  note: -m(t)
  note: m(t)
  note: S2(t)
  note: S1(t)
  Input Signal : Inport
  Carrier Signal : Inport  Port=2
  -S2(t) : Product
  Add : Sum
  Add1 : Sum
  Add2 : Sum
  Constant : Constant
  Constant1 : Constant  Value=-1
  Constant2 : Constant
  Constant3 : Constant  Value=-1
  Product1 : Product
  S1(t) : Product
  S2(t) : Product
  DSBSC : Outport
  wires:
  Product1/1 -> Add1/1
  Add/1 -> S1(t)/1
  Constant3/1 -> -S2(t)/2
  Constant2/1 -> Add1/2
  S2(t)/1 -> -S2(t)/1
  Carrier Signal/1 -> S1(t)/2, S2(t)/1
  Constant/1 -> Add/2
  Add1/1 -> S2(t)/2
  Constant1/1 -> Product1/2
  -S2(t)/1 -> Add2/2
  S1(t)/1 -> Add2/1
  Input Signal/1 -> Product1/1, Add/1
  Add2/1 -> DSBSC/1

== system signal_tranmission/SSB Modulator65/Balanced Modulator ==
  note: -S2(t)
  note: S1(t)
  note: -m(t)
  note: m(t)
  note: S2(t)
  note: S1(t)
  Input Signal : Inport
  Carrier Signal : Inport  Port=2
  -S2(t) : Product
  Add : Sum
  Add1 : Sum
  Add2 : Sum
  Constant : Constant
  Constant1 : Constant  Value=-1
  Constant2 : Constant
  Constant3 : Constant  Value=-1
  Product1 : Product
  S1(t) : Product
  S2(t) : Product
  DSBSC : Outport
  wires:
  Product1/1 -> Add1/1
  Add/1 -> S1(t)/1
  Constant3/1 -> -S2(t)/2
  Constant2/1 -> Add1/2
  S2(t)/1 -> -S2(t)/1
  Carrier Signal/1 -> S1(t)/2, S2(t)/1
  Constant/1 -> Add/2
  Add1/1 -> S2(t)/2
  Constant1/1 -> Product1/2
  -S2(t)/1 -> Add2/2
  S1(t)/1 -> Add2/1
  Input Signal/1 -> Product1/1, Add/1
  Add2/1 -> DSBSC/1

== system signal_tranmission/SSB Modulator66/Balanced Modulator ==
  note: -S2(t)
  note: S1(t)
  note: -m(t)
  note: m(t)
  note: S2(t)
  note: S1(t)
  Input Signal : Inport
  Carrier Signal : Inport  Port=2
  -S2(t) : Product
  Add : Sum
  Add1 : Sum
  Add2 : Sum
  Constant : Constant
  Constant1 : Constant  Value=-1
  Constant2 : Constant
  Constant3 : Constant  Value=-1
  Product1 : Product
  S1(t) : Product
  S2(t) : Product
  DSBSC : Outport
  wires:
  Product1/1 -> Add1/1
  Add/1 -> S1(t)/1
  Constant3/1 -> -S2(t)/2
  Constant2/1 -> Add1/2
  S2(t)/1 -> -S2(t)/1
  Carrier Signal/1 -> S1(t)/2, S2(t)/1
  Constant/1 -> Add/2
  Add1/1 -> S2(t)/2
  Constant1/1 -> Product1/2
  -S2(t)/1 -> Add2/2
  S1(t)/1 -> Add2/1
  Input Signal/1 -> Product1/1, Add/1
  Add2/1 -> DSBSC/1

== system signal_tranmission/SSB Modulator67/Balanced Modulator ==
  note: -S2(t)
  note: S1(t)
  note: -m(t)
  note: m(t)
  note: S2(t)
  note: S1(t)
  Input Signal : Inport
  Carrier Signal : Inport  Port=2
  -S2(t) : Product
  Add : Sum
  Add1 : Sum
  Add2 : Sum
  Constant : Constant
  Constant1 : Constant  Value=-1
  Constant2 : Constant
  Constant3 : Constant  Value=-1
  Product1 : Product
  S1(t) : Product
  S2(t) : Product
  DSBSC : Outport
  wires:
  Product1/1 -> Add1/1
  Add/1 -> S1(t)/1
  Constant3/1 -> -S2(t)/2
  Constant2/1 -> Add1/2
  S2(t)/1 -> -S2(t)/1
  Carrier Signal/1 -> S1(t)/2, S2(t)/1
  Constant/1 -> Add/2
  Add1/1 -> S2(t)/2
  Constant1/1 -> Product1/2
  -S2(t)/1 -> Add2/2
  S1(t)/1 -> Add2/1
  Input Signal/1 -> Product1/1, Add/1
  Add2/1 -> DSBSC/1

== system signal_tranmission/SSB Modulator68/Balanced Modulator ==
  note: -S2(t)
  note: S1(t)
  note: -m(t)
  note: m(t)
  note: S2(t)
  note: S1(t)
  Input Signal : Inport
  Carrier Signal : Inport  Port=2
  -S2(t) : Product
  Add : Sum
  Add1 : Sum
  Add2 : Sum
  Constant : Constant
  Constant1 : Constant  Value=-1
  Constant2 : Constant
  Constant3 : Constant  Value=-1
  Product1 : Product
  S1(t) : Product
  S2(t) : Product
  DSBSC : Outport
  wires:
  Product1/1 -> Add1/1
  Add/1 -> S1(t)/1
  Constant3/1 -> -S2(t)/2
  Constant2/1 -> Add1/2
  S2(t)/1 -> -S2(t)/1
  Carrier Signal/1 -> S1(t)/2, S2(t)/1
  Constant/1 -> Add/2
  Add1/1 -> S2(t)/2
  Constant1/1 -> Product1/2
  -S2(t)/1 -> Add2/2
  S1(t)/1 -> Add2/1
  Input Signal/1 -> Product1/1, Add/1
  Add2/1 -> DSBSC/1

== system signal_tranmission/SSB Modulator69/Balanced Modulator ==
  note: -S2(t)
  note: S1(t)
  note: -m(t)
  note: m(t)
  note: S2(t)
  note: S1(t)
  Input Signal : Inport
  Carrier Signal : Inport  Port=2
  -S2(t) : Product
  Add : Sum
  Add1 : Sum
  Add2 : Sum
  Constant : Constant
  Constant1 : Constant  Value=-1
  Constant2 : Constant
  Constant3 : Constant  Value=-1
  Product1 : Product
  S1(t) : Product
  S2(t) : Product
  DSBSC : Outport
  wires:
  Product1/1 -> Add1/1
  Add/1 -> S1(t)/1
  Constant3/1 -> -S2(t)/2
  Constant2/1 -> Add1/2
  S2(t)/1 -> -S2(t)/1
  Carrier Signal/1 -> S1(t)/2, S2(t)/1
  Constant/1 -> Add/2
  Add1/1 -> S2(t)/2
  Constant1/1 -> Product1/2
  -S2(t)/1 -> Add2/2
  S1(t)/1 -> Add2/1
  Input Signal/1 -> Product1/1, Add/1
  Add2/1 -> DSBSC/1

== system signal_tranmission/SSB Modulator7/Balanced Modulator ==
  note: -S2(t)
  note: S1(t)
  note: -m(t)
  note: m(t)
  note: S2(t)
  note: S1(t)
  Input Signal : Inport
  Carrier Signal : Inport  Port=2
  -S2(t) : Product
  Add : Sum
  Add1 : Sum
  Add2 : Sum
  Constant : Constant
  Constant1 : Constant  Value=-1
  Constant2 : Constant
  Constant3 : Constant  Value=-1
  Product1 : Product
  S1(t) : Product
  S2(t) : Product
  DSBSC : Outport
  wires:
  Product1/1 -> Add1/1
  Add/1 -> S1(t)/1
  Constant3/1 -> -S2(t)/2
  Constant2/1 -> Add1/2
  S2(t)/1 -> -S2(t)/1
  Carrier Signal/1 -> S1(t)/2, S2(t)/1
  Constant/1 -> Add/2
  Add1/1 -> S2(t)/2
  Constant1/1 -> Product1/2
  -S2(t)/1 -> Add2/2
  S1(t)/1 -> Add2/1
  Input Signal/1 -> Product1/1, Add/1
  Add2/1 -> DSBSC/1

== system signal_tranmission/SSB Modulator70/Balanced Modulator ==
  note: -S2(t)
  note: S1(t)
  note: -m(t)
  note: m(t)
  note: S2(t)
  note: S1(t)
  Input Signal : Inport
  Carrier Signal : Inport  Port=2
  -S2(t) : Product
  Add : Sum
  Add1 : Sum
  Add2 : Sum
  Constant : Constant
  Constant1 : Constant  Value=-1
  Constant2 : Constant
  Constant3 : Constant  Value=-1
  Product1 : Product
  S1(t) : Product
  S2(t) : Product
  DSBSC : Outport
  wires:
  Product1/1 -> Add1/1
  Add/1 -> S1(t)/1
  Constant3/1 -> -S2(t)/2
  Constant2/1 -> Add1/2
  S2(t)/1 -> -S2(t)/1
  Carrier Signal/1 -> S1(t)/2, S2(t)/1
  Constant/1 -> Add/2
  Add1/1 -> S2(t)/2
  Constant1/1 -> Product1/2
  -S2(t)/1 -> Add2/2
  S1(t)/1 -> Add2/1
  Input Signal/1 -> Product1/1, Add/1
  Add2/1 -> DSBSC/1

== system signal_tranmission/SSB Modulator71/Balanced Modulator ==
  note: -S2(t)
  note: S1(t)
  note: -m(t)
  note: m(t)
  note: S2(t)
  note: S1(t)
  Input Signal : Inport
  Carrier Signal : Inport  Port=2
  -S2(t) : Product
  Add : Sum
  Add1 : Sum
  Add2 : Sum
  Constant : Constant
  Constant1 : Constant  Value=-1
  Constant2 : Constant
  Constant3 : Constant  Value=-1
  Product1 : Product
  S1(t) : Product
  S2(t) : Product
  DSBSC : Outport
  wires:
  Product1/1 -> Add1/1
  Add/1 -> S1(t)/1
  Constant3/1 -> -S2(t)/2
  Constant2/1 -> Add1/2
  S2(t)/1 -> -S2(t)/1
  Carrier Signal/1 -> S1(t)/2, S2(t)/1
  Constant/1 -> Add/2
  Add1/1 -> S2(t)/2
  Constant1/1 -> Product1/2
  -S2(t)/1 -> Add2/2
  S1(t)/1 -> Add2/1
  Input Signal/1 -> Product1/1, Add/1
  Add2/1 -> DSBSC/1

== system signal_tranmission/SSB Modulator72/Balanced Modulator ==
  note: -S2(t)
  note: S1(t)
  note: -m(t)
  note: m(t)
  note: S2(t)
  note: S1(t)
  Input Signal : Inport
  Carrier Signal : Inport  Port=2
  -S2(t) : Product
  Add : Sum
  Add1 : Sum
  Add2 : Sum
  Constant : Constant
  Constant1 : Constant  Value=-1
  Constant2 : Constant
  Constant3 : Constant  Value=-1
  Product1 : Product
  S1(t) : Product
  S2(t) : Product
  DSBSC : Outport
  wires:
  Product1/1 -> Add1/1
  Add/1 -> S1(t)/1
  Constant3/1 -> -S2(t)/2
  Constant2/1 -> Add1/2
  S2(t)/1 -> -S2(t)/1
  Carrier Signal/1 -> S1(t)/2, S2(t)/1
  Constant/1 -> Add/2
  Add1/1 -> S2(t)/2
  Constant1/1 -> Product1/2
  -S2(t)/1 -> Add2/2
  S1(t)/1 -> Add2/1
  Input Signal/1 -> Product1/1, Add/1
  Add2/1 -> DSBSC/1

== system signal_tranmission/SSB Modulator73/Balanced Modulator ==
  note: -S2(t)
  note: S1(t)
  note: -m(t)
  note: m(t)
  note: S2(t)
  note: S1(t)
  Input Signal : Inport
  Carrier Signal : Inport  Port=2
  -S2(t) : Product
  Add : Sum
  Add1 : Sum
  Add2 : Sum
  Constant : Constant
  Constant1 : Constant  Value=-1
  Constant2 : Constant
  Constant3 : Constant  Value=-1
  Product1 : Product
  S1(t) : Product
  S2(t) : Product
  DSBSC : Outport
  wires:
  Product1/1 -> Add1/1
  Add/1 -> S1(t)/1
  Constant3/1 -> -S2(t)/2
  Constant2/1 -> Add1/2
  S2(t)/1 -> -S2(t)/1
  Carrier Signal/1 -> S1(t)/2, S2(t)/1
  Constant/1 -> Add/2
  Add1/1 -> S2(t)/2
  Constant1/1 -> Product1/2
  -S2(t)/1 -> Add2/2
  S1(t)/1 -> Add2/1
  Input Signal/1 -> Product1/1, Add/1
  Add2/1 -> DSBSC/1

== system signal_tranmission/SSB Modulator74/Balanced Modulator ==
  note: -S2(t)
  note: S1(t)
  note: -m(t)
  note: m(t)
  note: S2(t)
  note: S1(t)
  Input Signal : Inport
  Carrier Signal : Inport  Port=2
  -S2(t) : Product
  Add : Sum
  Add1 : Sum
  Add2 : Sum
  Constant : Constant
  Constant1 : Constant  Value=-1
  Constant2 : Constant
  Constant3 : Constant  Value=-1
  Product1 : Product
  S1(t) : Product
  S2(t) : Product
  DSBSC : Outport
  wires:
  Product1/1 -> Add1/1
  Add/1 -> S1(t)/1
  Constant3/1 -> -S2(t)/2
  Constant2/1 -> Add1/2
  S2(t)/1 -> -S2(t)/1
  Carrier Signal/1 -> S1(t)/2, S2(t)/1
  Constant/1 -> Add/2
  Add1/1 -> S2(t)/2
  Constant1/1 -> Product1/2
  -S2(t)/1 -> Add2/2
  S1(t)/1 -> Add2/1
  Input Signal/1 -> Product1/1, Add/1
  Add2/1 -> DSBSC/1

== system signal_tranmission/SSB Modulator75/Balanced Modulator ==
  note: -S2(t)
  note: S1(t)
  note: -m(t)
  note: m(t)
  note: S2(t)
  note: S1(t)
  Input Signal : Inport
  Carrier Signal : Inport  Port=2
  -S2(t) : Product
  Add : Sum
  Add1 : Sum
  Add2 : Sum
  Constant : Constant
  Constant1 : Constant  Value=-1
  Constant2 : Constant
  Constant3 : Constant  Value=-1
  Product1 : Product
  S1(t) : Product
  S2(t) : Product
  DSBSC : Outport
  wires:
  Product1/1 -> Add1/1
  Add/1 -> S1(t)/1
  Constant3/1 -> -S2(t)/2
  Constant2/1 -> Add1/2
  S2(t)/1 -> -S2(t)/1
  Carrier Signal/1 -> S1(t)/2, S2(t)/1
  Constant/1 -> Add/2
  Add1/1 -> S2(t)/2
  Constant1/1 -> Product1/2
  -S2(t)/1 -> Add2/2
  S1(t)/1 -> Add2/1
  Input Signal/1 -> Product1/1, Add/1
  Add2/1 -> DSBSC/1

== system signal_tranmission/SSB Modulator76/Balanced Modulator ==
  note: -S2(t)
  note: S1(t)
  note: -m(t)
  note: m(t)
  note: S2(t)
  note: S1(t)
  Input Signal : Inport
  Carrier Signal : Inport  Port=2
  -S2(t) : Product
  Add : Sum
  Add1 : Sum
  Add2 : Sum
  Constant : Constant
  Constant1 : Constant  Value=-1
  Constant2 : Constant
  Constant3 : Constant  Value=-1
  Product1 : Product
  S1(t) : Product
  S2(t) : Product
  DSBSC : Outport
  wires:
  Product1/1 -> Add1/1
  Add/1 -> S1(t)/1
  Constant3/1 -> -S2(t)/2
  Constant2/1 -> Add1/2
  S2(t)/1 -> -S2(t)/1
  Carrier Signal/1 -> S1(t)/2, S2(t)/1
  Constant/1 -> Add/2
  Add1/1 -> S2(t)/2
  Constant1/1 -> Product1/2
  -S2(t)/1 -> Add2/2
  S1(t)/1 -> Add2/1
  Input Signal/1 -> Product1/1, Add/1
  Add2/1 -> DSBSC/1

== system signal_tranmission/SSB Modulator77/Balanced Modulator ==
  note: -S2(t)
  note: S1(t)
  note: -m(t)
  note: m(t)
  note: S2(t)
  note: S1(t)
  Input Signal : Inport
  Carrier Signal : Inport  Port=2
  -S2(t) : Product
  Add : Sum
  Add1 : Sum
  Add2 : Sum
  Constant : Constant
  Constant1 : Constant  Value=-1
  Constant2 : Constant
  Constant3 : Constant  Value=-1
  Product1 : Product
  S1(t) : Product
  S2(t) : Product
  DSBSC : Outport
  wires:
  Product1/1 -> Add1/1
  Add/1 -> S1(t)/1
  Constant3/1 -> -S2(t)/2
  Constant2/1 -> Add1/2
  S2(t)/1 -> -S2(t)/1
  Carrier Signal/1 -> S1(t)/2, S2(t)/1
  Constant/1 -> Add/2
  Add1/1 -> S2(t)/2
  Constant1/1 -> Product1/2
  -S2(t)/1 -> Add2/2
  S1(t)/1 -> Add2/1
  Input Signal/1 -> Product1/1, Add/1
  Add2/1 -> DSBSC/1

== system signal_tranmission/SSB Modulator78/Balanced Modulator ==
  note: -S2(t)
  note: S1(t)
  note: -m(t)
  note: m(t)
  note: S2(t)
  note: S1(t)
  Input Signal : Inport
  Carrier Signal : Inport  Port=2
  -S2(t) : Product
  Add : Sum
  Add1 : Sum
  Add2 : Sum
  Constant : Constant
  Constant1 : Constant  Value=-1
  Constant2 : Constant
  Constant3 : Constant  Value=-1
  Product1 : Product
  S1(t) : Product
  S2(t) : Product
  DSBSC : Outport
  wires:
  Product1/1 -> Add1/1
  Add/1 -> S1(t)/1
  Constant3/1 -> -S2(t)/2
  Constant2/1 -> Add1/2
  S2(t)/1 -> -S2(t)/1
  Carrier Signal/1 -> S1(t)/2, S2(t)/1
  Constant/1 -> Add/2
  Add1/1 -> S2(t)/2
  Constant1/1 -> Product1/2
  -S2(t)/1 -> Add2/2
  S1(t)/1 -> Add2/1
  Input Signal/1 -> Product1/1, Add/1
  Add2/1 -> DSBSC/1
